simulink model "m_model"  (R2019a)
settings: Solver=VariableStepAuto  StartTime=0.0  StopTime=10.0  RelTol=1e-3
undefined symbols (not defined in the file or in its folder): K, lambda
settings Model: Creator=rache  LastModifiedBy=rache

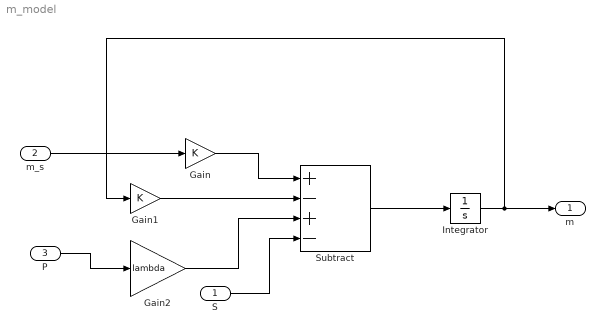
== system m_model ==
  S : Inport
  m_s : Inport  Port=2
  P : Inport  Port=3
  Gain : Gain  Gain=K
  Gain1 : Gain  Gain=K
  Gain2 : Gain  Gain=lambda
  Integrator : Integrator
  Subtract : Sum  Inputs=+-+-
  m : Outport
  wires:
  Gain/1 -> Subtract/1
  Gain1/1 -> Subtract/2
  Gain2/1 -> Subtract/3
  S/1 -> Subtract/4
  Subtract/1 -> Integrator/1
  Integrator/1 -> m/1, Gain1/1
  m_s/1 -> Gain/1
  P/1 -> Gain2/1
